simulink model "RST"  (R2021a)
settings: Solver=VariableStepAuto  StartTime=0.0  StopTime=10  RelTol=1e-3
settings Model: Creator=lenovo  LastModifiedBy=lenovo

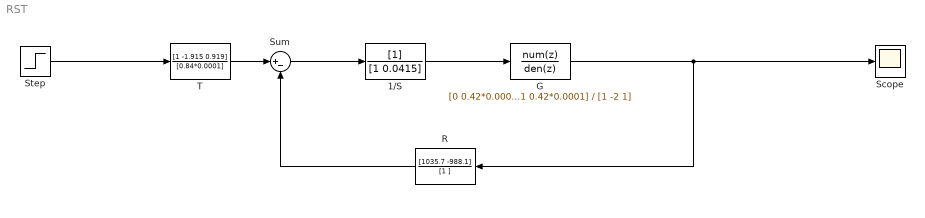
== system RST ==
  1/S : DiscreteFilter  Denominator=[1 0.0415]
  G : DiscreteFilter  Numerator=[0 0.42*0.0001 0.42*0.0001]  Denominator=[1 -2 1]
  R : DiscreteFilter  Numerator=[1035.7 -988.1]  Denominator=[1 ]
  Scope : Scope
  Step : Step  Time=0  SampleTime=0
  Sum : Sum  Inputs=|+-
  T : DiscreteFilter  Numerator=[1 -1.915 0.919]  Denominator=[0.84*0.0001]
  wires:
  R/1 -> Sum/2
  Step/1 -> T/1
  Sum/1 -> 1/S/1
  1/S/1 -> G/1
  T/1 -> Sum/1
  G/1 -> R/1, Scope/1
